simulink model "Combined_Pade_Model_D"  (R2020b)
settings: Solver=VariableStepAuto  StartTime=0.0  StopTime=t_final  MaxStep=0.1  RelTol=1e-3
values from neighbouring files (symbols this model uses):
  c = evalin('base','c')    [output_T.m]    (also in output_V.m; state_eqns_combined_2_n.m; state_eqns_combined_3_n.m; state_eqns_combined_4_n.m)
  p2 = evalin('base','p2')    [output_C_2.m]    (also in state_eqns_combined_2_n.m; state_eqns_combined_2_p.m)
  p3 = evalin('base','p3')    [output_C_3.m]    (also in state_eqns_combined_3_n.m; state_eqns_combined_3_p.m)
  p4 = evalin('base','p4')    [output_C_4.m]    (also in state_eqns_combined_4_n.m; state_eqns_combined_4_p.m)
  p5 = evalin('base','p5')    [output_C_5.m]    (also in state_eqns_combined_5_n.m; state_eqns_combined_5_p.m)
  p6 = evalin('base','p6')    [output_C_6.m]    (also in state_eqns_combined_6_n.m; state_eqns_combined_6_p.m)
  x1n_initial = 0    [Combined_Run_Model.m]
  x2n_initial = 0    [Combined_Run_Model.m]
  x2p_initial = 0    [Combined_Run_Model.m]
  x3n_initial = 0    [Combined_Run_Model.m]
  x3p_initial = 0    [Combined_Run_Model.m]
  x4n_initial = 0    [Combined_Run_Model.m]
  x4p_initial = 0    [Combined_Run_Model.m]
  x5n_initial = 0    [Combined_Run_Model.m]
  x5p_initial = 0    [Combined_Run_Model.m]
  x6n_initial = 0    [Combined_Run_Model.m]
  x6p_initial = 0    [Combined_Run_Model.m]
settings Model: Creator=moonjihoon  LastModifiedBy=moonjihoon

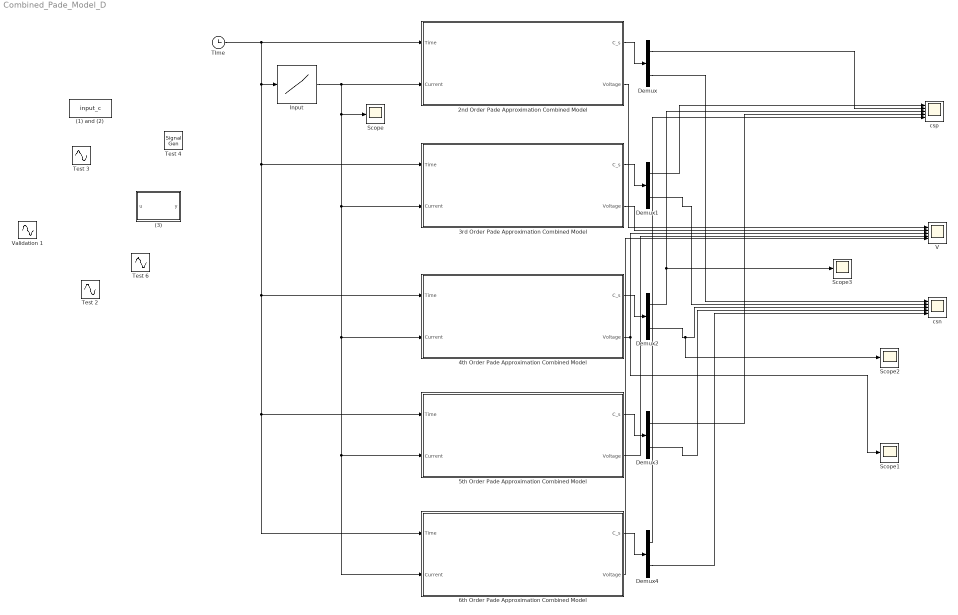
== system Combined_Pade_Model_D ==
  (1) and (2) : MATLABFcn  MATLABFcn=input_c
  (3) : MATLAB Function  TreatAsAtomicUnit=on
  2nd Order Pade Approximation Combined Model : Subsystem
  3rd Order Pade Approximation Combined Model : Subsystem
  4th Order Pade Approximation Combined Model : Subsystem
  5th Order Pade Approximation Combined Model : Subsystem
  6th Order Pade Approximation Combined Model : Subsystem
  Demux{,1..4} (5 alike) : Demux  Outputs=2
  Input : Lookup_n-D  NumberOfTableDimensions=1  BreakpointsForDimension1=t  Table=u  InternalRulePriority=Speed  RndMeth=Simplest  InputSameDT=on
  Scope{,1..3} (4 alike) : Scope
  TIme : Clock
  Test 2 : Sin  Amplitude=10  Frequency=0.005  Phase=3*pi/2  SampleTime=0
  Test 3 : Sin  Amplitude=6  Frequency=0.03  Phase=3*pi/2  SampleTime=0
  Test 4 : SignalGenerator  WaveForm=square  Amplitude=-4  Frequency=0.006  Units=rad/sec
  Test 6 : Sin  Amplitude=10  Frequency=0.005  SampleTime=0
  V : Scope  NumInputPorts=5
  Validation 1 : Sin  Amplitude=5  Frequency=0.02  SampleTime=0
  csn : Scope  NumInputPorts=5
  csp : Scope  NumInputPorts=5
  wires:
  TIme/1 -> Input/1, 6th Order Pade Approximation Combined Model/1(Time), 5th Order Pade Approximation Combined Model/1(Time), 4th Order Pade Approximation Combined Model/1(Time), 3rd Order Pade Approximation Combined Model/1(Time), 2nd Order Pade Approximation Combined Model/1(Time)
  Demux/2 -> csn/1
  Demux/1 -> csp/2
  2nd Order Pade Approximation Combined Model/1(C_s) -> Demux/1
  3rd Order Pade Approximation Combined Model/1(C_s) -> Demux1/1
  Demux1/2 -> csn/2
  Demux1/1 -> csp/1
  Input/1 -> Scope/1, 6th Order Pade Approximation Combined Model/2(Current), 5th Order Pade Approximation Combined Model/2(Current), 4th Order Pade Approximation Combined Model/2(Current), 3rd Order Pade Approximation Combined Model/2(Current), 2nd Order Pade Approximation Combined Model/2(Current)
  Demux2/2 -> Scope2/1, csn/3
  4th Order Pade Approximation Combined Model/1(C_s) -> Demux2/1
  Demux2/1 -> Scope3/1, csp/3
  Demux3/2 -> csn/4
  Demux3/1 -> csp/4
  5th Order Pade Approximation Combined Model/1(C_s) -> Demux3/1
  Demux4/1 -> csp/5
  Demux4/2 -> csn/5
  6th Order Pade Approximation Combined Model/1(C_s) -> Demux4/1
  2nd Order Pade Approximation Combined Model/2(Voltage) -> V/1
  3rd Order Pade Approximation Combined Model/2(Voltage) -> V/2
  4th Order Pade Approximation Combined Model/2(Voltage) -> Scope1/1, V/3
  5th Order Pade Approximation Combined Model/2(Voltage) -> V/4
  6th Order Pade Approximation Combined Model/2(Voltage) -> V/5

== system Combined_Pade_Model_D/2nd Order Pade Approximation Combined Model ==
  Time : Inport
  Current : Inport  Port=2
  Constant : Constant  Value=c.T_inf
  Negative Electrode1 : Subsystem
  OUtput Voltage : Subsystem
  Positive Electrode : Subsystem
  Surface Concentration1 : Subsystem
  C_s : Outport
  Voltage : Outport  Port=2
  wires:
  Time/1 -> Negative Electrode1/1(Time), OUtput Voltage/1(TIme), Surface Concentration1/1(TIme), Positive Electrode/1(TIme)
  Positive Electrode/1(X1,p) -> Surface Concentration1/2(X1,p)
  Positive Electrode/2(X2,p) -> Surface Concentration1/3(X2,p)
  Negative Electrode1/1(X1,n) -> Surface Concentration1/4(X1,n)
  Surface Concentration1/1(C_s) -> OUtput Voltage/3(C_s), C_s/1
  Negative Electrode1/2(X2,n) -> Surface Concentration1/5(X2,n)
  Current/1 -> Negative Electrode1/2(Current), OUtput Voltage/2(Current), Positive Electrode/2(Current)
  Negative Electrode1/3(x2_dot) -> Surface Concentration1/6(X2_dot)
  OUtput Voltage/1(Voltage) -> Voltage/1
  Constant/1 -> OUtput Voltage/4(T)

== system Combined_Pade_Model_D/3rd Order Pade Approximation Combined Model ==
  Time : Inport
  Current : Inport  Port=2
  Constant : Constant  Value=c.T_inf
  Negative Electrode : Subsystem
  OUtput Voltage : Subsystem
  Positive Electrode : Subsystem
  Surface Concentration1 : Subsystem
  C_s : Outport
  Voltage : Outport  Port=2
  wires:
  Time/1 -> OUtput Voltage/1(TIme), Negative Electrode/1(Time), Surface Concentration1/1(TIme), Positive Electrode/1(TIme)
  Current/1 -> Negative Electrode/2(Current), OUtput Voltage/2(Current), Positive Electrode/2(Current)
  Positive Electrode/1(X1,p) -> Surface Concentration1/2(X1,p)
  Positive Electrode/2(X2,p) -> Surface Concentration1/3(X2,p)
  Surface Concentration1/1(C_s) -> OUtput Voltage/3(C_s), C_s/1
  Positive Electrode/3(X3,p) -> Surface Concentration1/4(X3,p)
  Negative Electrode/1(X1,n) -> Surface Concentration1/5(X1,n)
  Negative Electrode/2(X2,n) -> Surface Concentration1/6(X2,n)
  Negative Electrode/3(X3,n) -> Surface Concentration1/7(X3,n)
  Negative Electrode/4(x3_dot) -> Surface Concentration1/8(X3_dot)
  OUtput Voltage/1(Voltage) -> Voltage/1
  Constant/1 -> OUtput Voltage/4(T)

== system Combined_Pade_Model_D/4th Order Pade Approximation Combined Model ==
  Time : Inport
  Current : Inport  Port=2
  Constant : Constant  Value=c.T_inf
  Negative Electrode : Subsystem
  OUtput Voltage : Subsystem
  Positive Electrode : Subsystem
  Surface Concentration1 : Subsystem
  C_s : Outport
  Voltage : Outport  Port=2
  wires:
  Time/1 -> Negative Electrode/1(Time), Positive Electrode/1(TIme), Surface Concentration1/1(TIme), OUtput Voltage/1(TIme)
  Current/1 -> OUtput Voltage/2(Current), Negative Electrode/2(Current), Positive Electrode/2(Current)
  Positive Electrode/1(X1,p) -> Surface Concentration1/2(X1,p)
  Positive Electrode/2(X2,p) -> Surface Concentration1/3(X2,p)
  Surface Concentration1/1(C_s) -> OUtput Voltage/3(C_s), C_s/1
  Positive Electrode/3(X3,p) -> Surface Concentration1/4(X3,p)
  Negative Electrode/5(x4_dot) -> Surface Concentration1/10(X4_dot)
  Positive Electrode/4(X4,p) -> Surface Concentration1/5(X4,p)
  Negative Electrode/1(X1,n) -> Surface Concentration1/6(X1,n)
  Negative Electrode/2(X2,n) -> Surface Concentration1/7(X2,n)
  Negative Electrode/3(X3,n) -> Surface Concentration1/8(X3,n)
  Negative Electrode/4(X4,n) -> Surface Concentration1/9(X4,n)
  OUtput Voltage/1(Voltage) -> Voltage/1
  Constant/1 -> OUtput Voltage/4(T)

== system Combined_Pade_Model_D/5th Order Pade Approximation Combined Model ==
  Time : Inport
  Current : Inport  Port=2
  Constant : Constant  Value=c.T_inf
  Negative Electrode : Subsystem
  OUtput Voltage : Subsystem
  Positive Electrode : Subsystem
  Surface Concentration1 : Subsystem
  C_s : Outport
  Voltage : Outport  Port=2
  wires:
  Time/1 -> Negative Electrode/1(Time), Positive Electrode/1(TIme), OUtput Voltage/1(TIme), Surface Concentration1/1(TIme)
  Current/1 -> Negative Electrode/2(Current), OUtput Voltage/2(Current), Positive Electrode/2(Current)
  Positive Electrode/1(X1,p) -> Surface Concentration1/2(X1,p)
  Positive Electrode/2(X2,p) -> Surface Concentration1/3(X2,p)
  Surface Concentration1/1(C_s) -> OUtput Voltage/3(C_s), C_s/1
  Positive Electrode/3(X3,p) -> Surface Concentration1/4(X3,p)
  Positive Electrode/4(X4,p) -> Surface Concentration1/5(X4,p)
  Positive Electrode/5(X5,p) -> Surface Concentration1/6(X5,p)
  Negative Electrode/1(X1,n) -> Surface Concentration1/7(X1,n)
  Negative Electrode/2(X2,n) -> Surface Concentration1/8(X2,n)
  Negative Electrode/3(X3,n) -> Surface Concentration1/9(X3,n)
  Negative Electrode/4(X4,n) -> Surface Concentration1/10(X4,n)
  Negative Electrode/5(X5,n) -> Surface Concentration1/11(X5,n)
  Negative Electrode/6(x5_dot) -> Surface Concentration1/12(X5_dot)
  OUtput Voltage/1(Voltage) -> Voltage/1
  Constant/1 -> OUtput Voltage/4(T)

== system Combined_Pade_Model_D/6th Order Pade Approximation Combined Model ==
  Time : Inport
  Current : Inport  Port=2
  Constant : Constant  Value=c.T_inf
  Negative Electrode : Subsystem
  OUtput Voltage : Subsystem
  Positive Electrode : Subsystem
  Surface Concentration1 : Subsystem
  C_s : Outport
  Voltage : Outport  Port=2
  wires:
  Time/1 -> Negative Electrode/1(Time), Positive Electrode/1(TIme), OUtput Voltage/1(TIme), Surface Concentration1/1(TIme)
  Current/1 -> OUtput Voltage/2(Current), Negative Electrode/2(Current), Positive Electrode/2(Current)
  Positive Electrode/1(X1,p) -> Surface Concentration1/2(X1,p)
  Positive Electrode/2(X2,p) -> Surface Concentration1/3(X2,p)
  Surface Concentration1/1(C_s) -> OUtput Voltage/3(C_s), C_s/1
  Positive Electrode/3(X3,p) -> Surface Concentration1/4(X3,p)
  Positive Electrode/4(X4,p) -> Surface Concentration1/5(X4,p)
  Positive Electrode/5(X5,p) -> Surface Concentration1/6(X5,p)
  Negative Electrode/1(X1,n) -> Surface Concentration1/8(X1,n)
  Negative Electrode/2(X2,n) -> Surface Concentration1/9(X2,n)
  Negative Electrode/3(X3,n) -> Surface Concentration1/10(X3,n)
  Negative Electrode/4(X4,n) -> Surface Concentration1/11(X4,n)
  Negative Electrode/5(X5,n) -> Surface Concentration1/12(X5,n)
  Negative Electrode/7(x6_dot) -> Surface Concentration1/14(X6_dot)
  Negative Electrode/6(X6,n) -> Surface Concentration1/13(X6,n)
  Positive Electrode/6(X6,p) -> Surface Concentration1/7(X6,p)
  OUtput Voltage/1(Voltage) -> Voltage/1
  Constant/1 -> OUtput Voltage/4(T)

== system Combined_Pade_Model_D/2nd Order Pade Approximation Combined Model/Negative Electrode1 ==
  Time : Inport
  Current : Inport  Port=2
  Dynamics : Subsystem
  X1,n : Outport
  X2,n : Outport  Port=2
  x2_dot : Outport  Port=3
  wires:
  Time/1 -> Dynamics/1(Time)
  Current/1 -> Dynamics/2(Current)
  Dynamics/1(X1,n) -> X1,n/1
  Dynamics/2(X2,n) -> X2,n/1
  Dynamics/3(x2_dot) -> x2_dot/1

== system Combined_Pade_Model_D/2nd Order Pade Approximation Combined Model/OUtput Voltage ==
  TIme : Inport
  Current : Inport  Port=2
  C_s : Inport  Port=3
  T : Inport  Port=4
  Interpreted MATLAB Function : MATLABFcn  MATLABFcn=output_V
  Mux : Mux
  Voltage : Outport
  wires:
  TIme/1 -> Mux/1
  Interpreted MATLAB Function/1 -> Voltage/1
  Mux/1 -> Interpreted MATLAB Function/1
  Current/1 -> Mux/2
  C_s/1 -> Mux/3
  T/1 -> Mux/4

== system Combined_Pade_Model_D/2nd Order Pade Approximation Combined Model/Positive Electrode ==
  TIme : Inport
  Current : Inport  Port=2
  Dynamics : Subsystem
  X1,p : Outport
  X2,p : Outport  Port=2
  wires:
  Current/1 -> Dynamics/2(Current)
  TIme/1 -> Dynamics/1(Time)
  Dynamics/1(X1,p) -> X1,p/1
  Dynamics/2(X2,p) -> X2,p/1

== system Combined_Pade_Model_D/2nd Order Pade Approximation Combined Model/Surface Concentration1 ==
  TIme : Inport
  X1,p : Inport  Port=2
  X2,p : Inport  Port=3
  X1,n : Inport  Port=4
  X2,n : Inport  Port=5
  X2_dot : Inport  Port=6
  Interpreted MATLAB Function : MATLABFcn  MATLABFcn=output_C_2
  Mux : Mux  Inputs=6
  C_s : Outport
  wires:
  Interpreted MATLAB Function/1 -> C_s/1
  Mux/1 -> Interpreted MATLAB Function/1
  X2,p/1 -> Mux/3
  TIme/1 -> Mux/1
  X1,p/1 -> Mux/2
  X1,n/1 -> Mux/4
  X2,n/1 -> Mux/5
  X2_dot/1 -> Mux/6

== system Combined_Pade_Model_D/3rd Order Pade Approximation Combined Model/Negative Electrode ==
  Time : Inport
  Current : Inport  Port=2
  Dynamics : Subsystem
  X1,n : Outport
  X2,n : Outport  Port=2
  X3,n : Outport  Port=3
  x3_dot : Outport  Port=4
  wires:
  Time/1 -> Dynamics/1(Time)
  Current/1 -> Dynamics/2(Current)
  Dynamics/1(X1,n) -> X1,n/1
  Dynamics/2(X2,n) -> X2,n/1
  Dynamics/3(X2,n1) -> X3,n/1
  Dynamics/4(x3_dot) -> x3_dot/1

== system Combined_Pade_Model_D/3rd Order Pade Approximation Combined Model/OUtput Voltage ==
  TIme : Inport
  Current : Inport  Port=2
  C_s : Inport  Port=3
  T : Inport  Port=4
  Interpreted MATLAB Function : MATLABFcn  MATLABFcn=output_V
  Mux : Mux
  Voltage : Outport
  wires:
  TIme/1 -> Mux/1
  Interpreted MATLAB Function/1 -> Voltage/1
  Mux/1 -> Interpreted MATLAB Function/1
  Current/1 -> Mux/2
  C_s/1 -> Mux/3
  T/1 -> Mux/4

== system Combined_Pade_Model_D/3rd Order Pade Approximation Combined Model/Positive Electrode ==
  TIme : Inport
  Current : Inport  Port=2
  Dynamics : Subsystem
  X1,p : Outport
  X2,p : Outport  Port=2
  X3,p : Outport  Port=3
  wires:
  Current/1 -> Dynamics/2(Current)
  TIme/1 -> Dynamics/1(Time)
  Dynamics/1(X1,p) -> X1,p/1
  Dynamics/2(X2,p) -> X2,p/1
  Dynamics/3(X3,p) -> X3,p/1

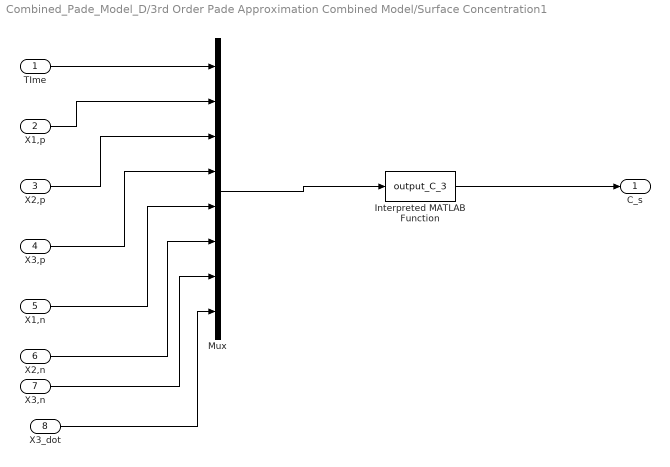
== system Combined_Pade_Model_D/3rd Order Pade Approximation Combined Model/Surface Concentration1 ==
  TIme : Inport
  X1,p : Inport  Port=2
  X2,p : Inport  Port=3
  X3,p : Inport  Port=4
  X1,n : Inport  Port=5
  X2,n : Inport  Port=6
  X3,n : Inport  Port=7
  X3_dot : Inport  Port=8
  Interpreted MATLAB Function : MATLABFcn  MATLABFcn=output_C_3
  Mux : Mux  Inputs=8
  C_s : Outport
  wires:
  Interpreted MATLAB Function/1 -> C_s/1
  Mux/1 -> Interpreted MATLAB Function/1
  X2,p/1 -> Mux/3
  TIme/1 -> Mux/1
  X1,p/1 -> Mux/2
  X3,p/1 -> Mux/4
  X1,n/1 -> Mux/5
  X2,n/1 -> Mux/6
  X3,n/1 -> Mux/7
  X3_dot/1 -> Mux/8

== system Combined_Pade_Model_D/4th Order Pade Approximation Combined Model/Negative Electrode ==
  Time : Inport
  Current : Inport  Port=2
  Dynamics : Subsystem
  X1,n : Outport
  X2,n : Outport  Port=2
  X3,n : Outport  Port=3
  X4,n : Outport  Port=4
  x4_dot : Outport  Port=5
  wires:
  Time/1 -> Dynamics/1(Time)
  Current/1 -> Dynamics/2(Current)
  Dynamics/1(X1,n) -> X1,n/1
  Dynamics/2(X2,n) -> X2,n/1
  Dynamics/3(X3,n) -> X3,n/1
  Dynamics/5(x4_dot) -> x4_dot/1
  Dynamics/4(X4,n) -> X4,n/1

== system Combined_Pade_Model_D/4th Order Pade Approximation Combined Model/OUtput Voltage ==
  TIme : Inport
  Current : Inport  Port=2
  C_s : Inport  Port=3
  T : Inport  Port=4
  Interpreted MATLAB Function : MATLABFcn  MATLABFcn=output_V
  Mux : Mux
  Voltage : Outport
  wires:
  TIme/1 -> Mux/1
  Interpreted MATLAB Function/1 -> Voltage/1
  Mux/1 -> Interpreted MATLAB Function/1
  Current/1 -> Mux/2
  C_s/1 -> Mux/3
  T/1 -> Mux/4

== system Combined_Pade_Model_D/4th Order Pade Approximation Combined Model/Positive Electrode ==
  TIme : Inport
  Current : Inport  Port=2
  Dynamics : Subsystem
  X1,p : Outport
  X2,p : Outport  Port=2
  X3,p : Outport  Port=3
  X4,p : Outport  Port=4
  wires:
  Current/1 -> Dynamics/2(Current)
  TIme/1 -> Dynamics/1(Time)
  Dynamics/1(X1,p) -> X1,p/1
  Dynamics/2(X2,p) -> X2,p/1
  Dynamics/3(X3,p) -> X3,p/1
  Dynamics/4(X4,p) -> X4,p/1

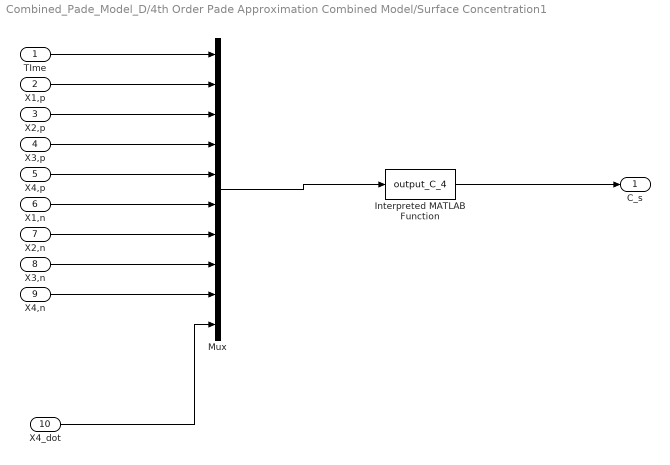
== system Combined_Pade_Model_D/4th Order Pade Approximation Combined Model/Surface Concentration1 ==
  TIme : Inport
  X1,p : Inport  Port=2
  X2,p : Inport  Port=3
  X3,p : Inport  Port=4
  X4,p : Inport  Port=5
  X1,n : Inport  Port=6
  X2,n : Inport  Port=7
  X3,n : Inport  Port=8
  X4,n : Inport  Port=9
  X4_dot : Inport  Port=10
  Interpreted MATLAB Function : MATLABFcn  MATLABFcn=output_C_4
  Mux : Mux  Inputs=10
  C_s : Outport
  wires:
  Interpreted MATLAB Function/1 -> C_s/1
  Mux/1 -> Interpreted MATLAB Function/1
  X2,p/1 -> Mux/3
  TIme/1 -> Mux/1
  X1,p/1 -> Mux/2
  X3,p/1 -> Mux/4
  X4,p/1 -> Mux/5
  X1,n/1 -> Mux/6
  X2,n/1 -> Mux/7
  X4_dot/1 -> Mux/10
  X3,n/1 -> Mux/8
  X4,n/1 -> Mux/9

== system Combined_Pade_Model_D/5th Order Pade Approximation Combined Model/Negative Electrode ==
  Time : Inport
  Current : Inport  Port=2
  Dynamics : Subsystem
  X1,n : Outport
  X2,n : Outport  Port=2
  X3,n : Outport  Port=3
  X4,n : Outport  Port=4
  X5,n : Outport  Port=5
  x5_dot : Outport  Port=6
  wires:
  Time/1 -> Dynamics/1(Time)
  Current/1 -> Dynamics/2(Current)
  Dynamics/1(X1,n) -> X1,n/1
  Dynamics/2(X2,n) -> X2,n/1
  Dynamics/3(X3,n) -> X3,n/1
  Dynamics/6(x5_dot) -> x5_dot/1
  Dynamics/4(X4,n) -> X4,n/1
  Dynamics/5(X5,n) -> X5,n/1

== system Combined_Pade_Model_D/5th Order Pade Approximation Combined Model/OUtput Voltage ==
  TIme : Inport
  Current : Inport  Port=2
  C_s : Inport  Port=3
  T : Inport  Port=4
  Interpreted MATLAB Function : MATLABFcn  MATLABFcn=output_V
  Mux : Mux
  Voltage : Outport
  wires:
  TIme/1 -> Mux/1
  Interpreted MATLAB Function/1 -> Voltage/1
  Mux/1 -> Interpreted MATLAB Function/1
  Current/1 -> Mux/2
  C_s/1 -> Mux/3
  T/1 -> Mux/4

== system Combined_Pade_Model_D/5th Order Pade Approximation Combined Model/Positive Electrode ==
  TIme : Inport
  Current : Inport  Port=2
  Dynamics : Subsystem
  X1,p : Outport
  X2,p : Outport  Port=2
  X3,p : Outport  Port=3
  X4,p : Outport  Port=4
  X5,p : Outport  Port=5
  wires:
  Current/1 -> Dynamics/2(Current)
  TIme/1 -> Dynamics/1(Time)
  Dynamics/1(X1,p) -> X1,p/1
  Dynamics/2(X2,p) -> X2,p/1
  Dynamics/3(X3,p) -> X3,p/1
  Dynamics/4(X4,p) -> X4,p/1
  Dynamics/5(X5,p) -> X5,p/1

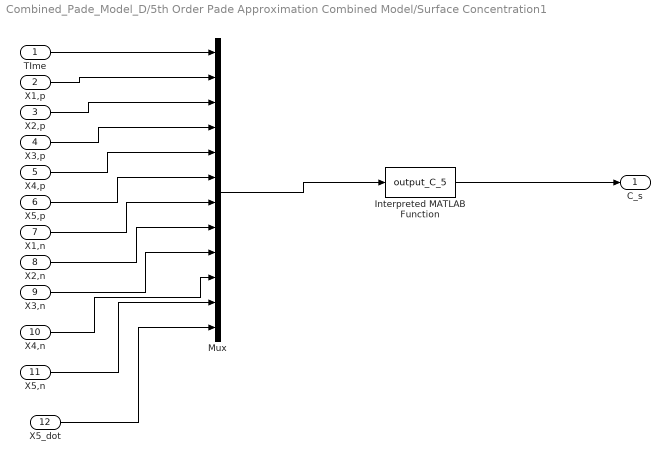
== system Combined_Pade_Model_D/5th Order Pade Approximation Combined Model/Surface Concentration1 ==
  TIme : Inport
  X1,p : Inport  Port=2
  X2,p : Inport  Port=3
  X3,p : Inport  Port=4
  X4,p : Inport  Port=5
  X5,p : Inport  Port=6
  X1,n : Inport  Port=7
  X2,n : Inport  Port=8
  X3,n : Inport  Port=9
  X4,n : Inport  Port=10
  X5,n : Inport  Port=11
  X5_dot : Inport  Port=12
  Interpreted MATLAB Function : MATLABFcn  MATLABFcn=output_C_5
  Mux : Mux  Inputs=12
  C_s : Outport
  wires:
  Interpreted MATLAB Function/1 -> C_s/1
  Mux/1 -> Interpreted MATLAB Function/1
  X2,p/1 -> Mux/3
  TIme/1 -> Mux/1
  X1,p/1 -> Mux/2
  X3,p/1 -> Mux/4
  X4,p/1 -> Mux/5
  X5,p/1 -> Mux/6
  X1,n/1 -> Mux/7
  X2,n/1 -> Mux/8
  X3,n/1 -> Mux/9
  X5_dot/1 -> Mux/12
  X4,n/1 -> Mux/10
  X5,n/1 -> Mux/11

== system Combined_Pade_Model_D/6th Order Pade Approximation Combined Model/Negative Electrode ==
  Time : Inport
  Current : Inport  Port=2
  Dynamics : Subsystem
  X1,n : Outport
  X2,n : Outport  Port=2
  X3,n : Outport  Port=3
  X4,n : Outport  Port=4
  X5,n : Outport  Port=5
  X6,n : Outport  Port=6
  x6_dot : Outport  Port=7
  wires:
  Time/1 -> Dynamics/1(Time)
  Current/1 -> Dynamics/2(Current)
  Dynamics/1(X1,n) -> X1,n/1
  Dynamics/2(X2,n) -> X2,n/1
  Dynamics/3(X3,n) -> X3,n/1
  Dynamics/7(x6_dot) -> x6_dot/1
  Dynamics/4(X4,n) -> X4,n/1
  Dynamics/5(X5,n) -> X5,n/1
  Dynamics/6(X6,n) -> X6,n/1

== system Combined_Pade_Model_D/6th Order Pade Approximation Combined Model/OUtput Voltage ==
  TIme : Inport
  Current : Inport  Port=2
  C_s : Inport  Port=3
  T : Inport  Port=4
  Interpreted MATLAB Function : MATLABFcn  MATLABFcn=output_V
  Mux : Mux
  Voltage : Outport
  wires:
  TIme/1 -> Mux/1
  Interpreted MATLAB Function/1 -> Voltage/1
  Mux/1 -> Interpreted MATLAB Function/1
  Current/1 -> Mux/2
  C_s/1 -> Mux/3
  T/1 -> Mux/4

== system Combined_Pade_Model_D/6th Order Pade Approximation Combined Model/Positive Electrode ==
  TIme : Inport
  Current : Inport  Port=2
  Dynamics : Subsystem
  X1,p : Outport
  X2,p : Outport  Port=2
  X3,p : Outport  Port=3
  X4,p : Outport  Port=4
  X5,p : Outport  Port=5
  X6,p : Outport  Port=6
  wires:
  Current/1 -> Dynamics/2(Current)
  TIme/1 -> Dynamics/1(Time)
  Dynamics/1(X1,p) -> X1,p/1
  Dynamics/2(X2,p) -> X2,p/1
  Dynamics/3(X3,p) -> X3,p/1
  Dynamics/4(X4,p) -> X4,p/1
  Dynamics/5(X5,p) -> X5,p/1
  Dynamics/6(X6,p) -> X6,p/1

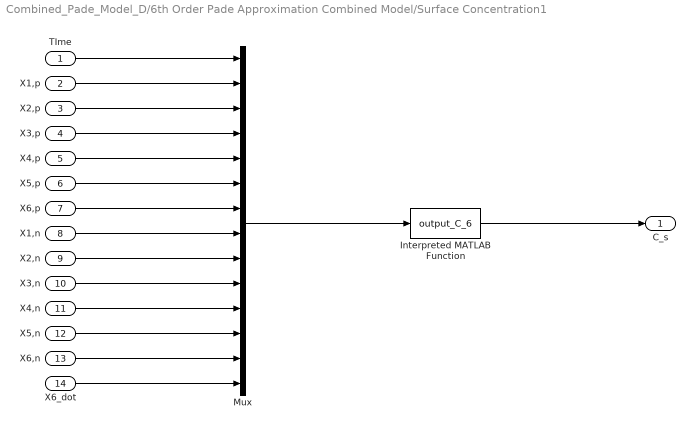
== system Combined_Pade_Model_D/6th Order Pade Approximation Combined Model/Surface Concentration1 ==
  TIme : Inport
  X1,p : Inport  Port=2
  X2,p : Inport  Port=3
  X3,p : Inport  Port=4
  X4,p : Inport  Port=5
  X5,p : Inport  Port=6
  X6,p : Inport  Port=7
  X1,n : Inport  Port=8
  X2,n : Inport  Port=9
  X3,n : Inport  Port=10
  X4,n : Inport  Port=11
  X5,n : Inport  Port=12
  X6,n : Inport  Port=13
  X6_dot : Inport  Port=14
  Interpreted MATLAB Function : MATLABFcn  MATLABFcn=output_C_6
  Mux : Mux  Inputs=14
  C_s : Outport
  wires:
  Interpreted MATLAB Function/1 -> C_s/1
  Mux/1 -> Interpreted MATLAB Function/1
  X6_dot/1 -> Mux/14
  TIme/1 -> Mux/1
  X1,p/1 -> Mux/2
  X2,p/1 -> Mux/3
  X3,p/1 -> Mux/4
  X4,p/1 -> Mux/5
  X5,p/1 -> Mux/6
  X6,p/1 -> Mux/7
  X1,n/1 -> Mux/8
  X2,n/1 -> Mux/9
  X3,n/1 -> Mux/10
  X4,n/1 -> Mux/11
  X5,n/1 -> Mux/12
  X6,n/1 -> Mux/13

== system Combined_Pade_Model_D/2nd Order Pade Approximation Combined Model/Negative Electrode1/Dynamics ==
  Time : Inport
  Current : Inport  Port=2
  Integrator : Integrator  InitialCondition=[x1n_initial;x2n_initial]
  Interpreted MATLAB Function : MATLABFcn  MATLABFcn=state_eqns_combined_2_n
  Mux : Mux  Inputs=3
  Selector : Selector  InputPortWidth=2  IndexOptions=Index vector (dialog)  Indices=[1]  OutputSizes=1
  Selector1 : Selector  InputPortWidth=2  IndexOptions=Index vector (dialog)  Indices=[2]  OutputSizes=1
  X1,n : Outport
  X2,n : Outport  Port=2
  x2_dot : Outport  Port=3
  wires:
  Current/1 -> Mux/2
  Time/1 -> Mux/1
  Selector/1 -> X1,n/1
  Selector1/1 -> X2,n/1
  Mux/1 -> Interpreted MATLAB Function/1
  Integrator/1 -> Mux/3, Selector1/1, Selector/1
  Interpreted MATLAB Function/1 -> x2_dot/1, Integrator/1

== system Combined_Pade_Model_D/2nd Order Pade Approximation Combined Model/Positive Electrode/Dynamics ==
  Time : Inport
  Current : Inport  Port=2
  Integrator : Integrator  InitialCondition=[p2.x1p_initial;x2p_initial]
  Interpreted MATLAB Function : MATLABFcn  MATLABFcn=state_eqns_combined_2_p
  Mux : Mux  Inputs=3
  Selector : Selector  InputPortWidth=2  IndexOptions=Index vector (dialog)  Indices=[1]  OutputSizes=1
  Selector1 : Selector  InputPortWidth=2  IndexOptions=Index vector (dialog)  Indices=[2]  OutputSizes=1
  X1,p : Outport
  X2,p : Outport  Port=2
  wires:
  Current/1 -> Mux/2
  Time/1 -> Mux/1
  Interpreted MATLAB Function/1 -> Integrator/1
  Selector/1 -> X1,p/1
  Selector1/1 -> X2,p/1
  Mux/1 -> Interpreted MATLAB Function/1
  Integrator/1 -> Mux/3, Selector1/1, Selector/1

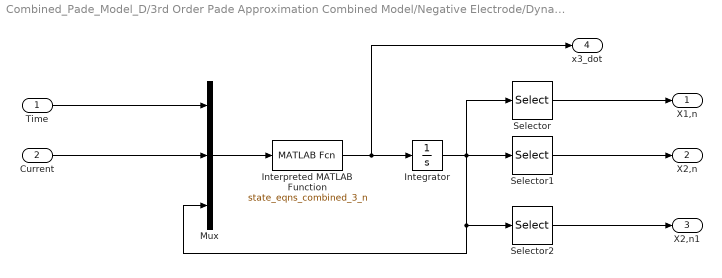
== system Combined_Pade_Model_D/3rd Order Pade Approximation Combined Model/Negative Electrode/Dynamics ==
  Time : Inport
  Current : Inport  Port=2
  Integrator : Integrator  InitialCondition=[x1n_initial;x2n_initial;x3n_initial]
  Interpreted MATLAB Function : MATLABFcn  MATLABFcn=state_eqns_combined_3_n
  Mux : Mux  Inputs=3
  Selector : Selector  InputPortWidth=3  IndexOptions=Index vector (dialog)  Indices=[1]  OutputSizes=1
  Selector1 : Selector  InputPortWidth=3  IndexOptions=Index vector (dialog)  Indices=[2]  OutputSizes=1
  Selector2 : Selector  InputPortWidth=3  IndexOptions=Index vector (dialog)  Indices=[3]  OutputSizes=1
  X1,n : Outport
  X2,n : Outport  Port=2
  X2,n1 : Outport  Port=3
  x3_dot : Outport  Port=4
  wires:
  Current/1 -> Mux/2
  Time/1 -> Mux/1
  Selector/1 -> X1,n/1
  Selector1/1 -> X2,n/1
  Mux/1 -> Interpreted MATLAB Function/1
  Selector2/1 -> X2,n1/1
  Integrator/1 -> Selector2/1, Mux/3, Selector1/1, Selector/1
  Interpreted MATLAB Function/1 -> x3_dot/1, Integrator/1

== system Combined_Pade_Model_D/3rd Order Pade Approximation Combined Model/Positive Electrode/Dynamics ==
  Time : Inport
  Current : Inport  Port=2
  Integrator : Integrator  InitialCondition=[p3.x1p_initial;x2p_initial;x3p_initial]
  Interpreted MATLAB Function : MATLABFcn  MATLABFcn=state_eqns_combined_3_p
  Mux : Mux  Inputs=3
  Selector : Selector  InputPortWidth=3  IndexOptions=Index vector (dialog)  Indices=[1]  OutputSizes=1
  Selector1 : Selector  InputPortWidth=3  IndexOptions=Index vector (dialog)  Indices=[2]  OutputSizes=1
  Selector2 : Selector  InputPortWidth=3  IndexOptions=Index vector (dialog)  Indices=[3]  OutputSizes=1
  X1,p : Outport
  X2,p : Outport  Port=2
  X3,p : Outport  Port=3
  wires:
  Current/1 -> Mux/2
  Time/1 -> Mux/1
  Interpreted MATLAB Function/1 -> Integrator/1
  Selector/1 -> X1,p/1
  Selector1/1 -> X2,p/1
  Mux/1 -> Interpreted MATLAB Function/1
  Integrator/1 -> Selector2/1, Mux/3, Selector1/1, Selector/1
  Selector2/1 -> X3,p/1

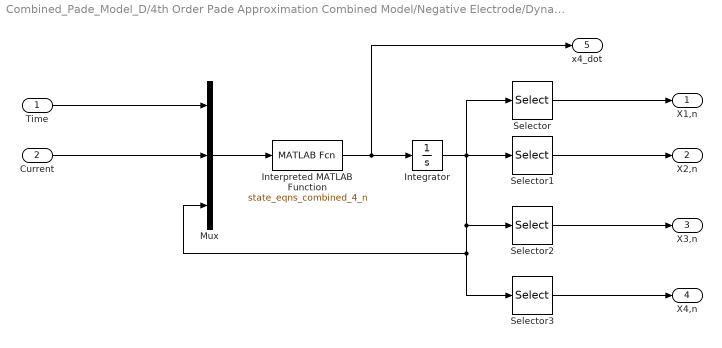
== system Combined_Pade_Model_D/4th Order Pade Approximation Combined Model/Negative Electrode/Dynamics ==
  Time : Inport
  Current : Inport  Port=2
  Integrator : Integrator  InitialCondition=[x1n_initial;x2n_initial;x3n_initial;x4n_initial]
  Interpreted MATLAB Function : MATLABFcn  MATLABFcn=state_eqns_combined_4_n
  Mux : Mux  Inputs=3
  Selector : Selector  InputPortWidth=4  IndexOptions=Index vector (dialog)  Indices=[1]  OutputSizes=1
  Selector1 : Selector  InputPortWidth=4  IndexOptions=Index vector (dialog)  Indices=[2]  OutputSizes=1
  Selector2 : Selector  InputPortWidth=4  IndexOptions=Index vector (dialog)  Indices=[3]  OutputSizes=1
  Selector3 : Selector  InputPortWidth=4  IndexOptions=Index vector (dialog)  Indices=[4]  OutputSizes=1
  X1,n : Outport
  X2,n : Outport  Port=2
  X3,n : Outport  Port=3
  X4,n : Outport  Port=4
  x4_dot : Outport  Port=5
  wires:
  Current/1 -> Mux/2
  Time/1 -> Mux/1
  Selector/1 -> X1,n/1
  Selector1/1 -> X2,n/1
  Mux/1 -> Interpreted MATLAB Function/1
  Selector2/1 -> X3,n/1
  Integrator/1 -> Selector2/1, Selector3/1, Mux/3, Selector1/1, Selector/1
  Interpreted MATLAB Function/1 -> x4_dot/1, Integrator/1
  Selector3/1 -> X4,n/1

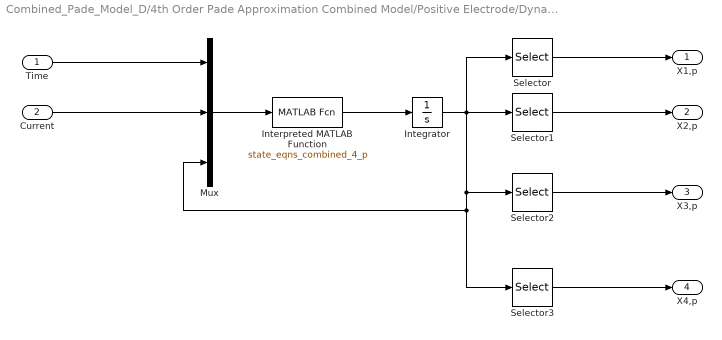
== system Combined_Pade_Model_D/4th Order Pade Approximation Combined Model/Positive Electrode/Dynamics ==
  Time : Inport
  Current : Inport  Port=2
  Integrator : Integrator  InitialCondition=[p4.x1p_initial;x2p_initial;x3p_initial;x4p_initial]
  Interpreted MATLAB Function : MATLABFcn  MATLABFcn=state_eqns_combined_4_p
  Mux : Mux  Inputs=3
  Selector : Selector  InputPortWidth=4  IndexOptions=Index vector (dialog)  Indices=[1]  OutputSizes=1
  Selector1 : Selector  InputPortWidth=4  IndexOptions=Index vector (dialog)  Indices=[2]  OutputSizes=1
  Selector2 : Selector  InputPortWidth=4  IndexOptions=Index vector (dialog)  Indices=[3]  OutputSizes=1
  Selector3 : Selector  InputPortWidth=4  IndexOptions=Index vector (dialog)  Indices=[4]  OutputSizes=1
  X1,p : Outport
  X2,p : Outport  Port=2
  X3,p : Outport  Port=3
  X4,p : Outport  Port=4
  wires:
  Current/1 -> Mux/2
  Time/1 -> Mux/1
  Interpreted MATLAB Function/1 -> Integrator/1
  Selector/1 -> X1,p/1
  Selector1/1 -> X2,p/1
  Mux/1 -> Interpreted MATLAB Function/1
  Selector2/1 -> X3,p/1
  Selector3/1 -> X4,p/1
  Integrator/1 -> Selector2/1, Selector3/1, Mux/3, Selector1/1, Selector/1

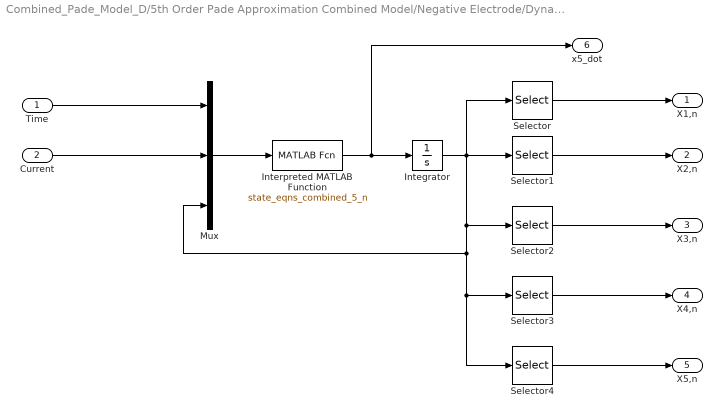
== system Combined_Pade_Model_D/5th Order Pade Approximation Combined Model/Negative Electrode/Dynamics ==
  Time : Inport
  Current : Inport  Port=2
  Integrator : Integrator  InitialCondition=[x1n_initial;x2n_initial;x3n_initial;x4n_initial;x5n_initial]
  Interpreted MATLAB Function : MATLABFcn  MATLABFcn=state_eqns_combined_5_n
  Mux : Mux  Inputs=3
  Selector : Selector  InputPortWidth=5  IndexOptions=Index vector (dialog)  Indices=[1]  OutputSizes=1
  Selector1 : Selector  InputPortWidth=5  IndexOptions=Index vector (dialog)  Indices=[2]  OutputSizes=1
  Selector2 : Selector  InputPortWidth=5  IndexOptions=Index vector (dialog)  Indices=[3]  OutputSizes=1
  Selector3 : Selector  InputPortWidth=5  IndexOptions=Index vector (dialog)  Indices=[4]  OutputSizes=1
  Selector4 : Selector  InputPortWidth=5  IndexOptions=Index vector (dialog)  Indices=[5]  OutputSizes=1
  X1,n : Outport
  X2,n : Outport  Port=2
  X3,n : Outport  Port=3
  X4,n : Outport  Port=4
  X5,n : Outport  Port=5
  x5_dot : Outport  Port=6
  wires:
  Current/1 -> Mux/2
  Time/1 -> Mux/1
  Selector/1 -> X1,n/1
  Selector1/1 -> X2,n/1
  Mux/1 -> Interpreted MATLAB Function/1
  Selector2/1 -> X3,n/1
  Interpreted MATLAB Function/1 -> x5_dot/1, Integrator/1
  Selector3/1 -> X4,n/1
  Selector4/1 -> X5,n/1
  Integrator/1 -> Selector2/1, Selector4/1, Selector3/1, Mux/3, Selector1/1, Selector/1

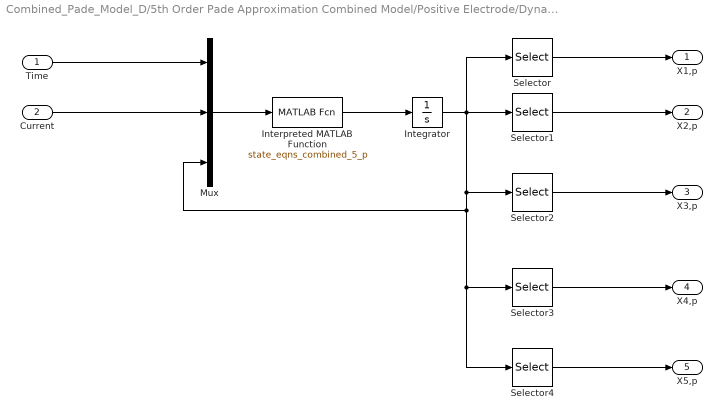
== system Combined_Pade_Model_D/5th Order Pade Approximation Combined Model/Positive Electrode/Dynamics ==
  Time : Inport
  Current : Inport  Port=2
  Integrator : Integrator  InitialCondition=[p5.x1p_initial;x2p_initial;x3p_initial;x4p_initial;x5p_initial]
  Interpreted MATLAB Function : MATLABFcn  MATLABFcn=state_eqns_combined_5_p
  Mux : Mux  Inputs=3
  Selector : Selector  InputPortWidth=5  IndexOptions=Index vector (dialog)  Indices=[1]  OutputSizes=1
  Selector1 : Selector  InputPortWidth=5  IndexOptions=Index vector (dialog)  Indices=[2]  OutputSizes=1
  Selector2 : Selector  InputPortWidth=5  IndexOptions=Index vector (dialog)  Indices=[3]  OutputSizes=1
  Selector3 : Selector  InputPortWidth=5  IndexOptions=Index vector (dialog)  Indices=[4]  OutputSizes=1
  Selector4 : Selector  InputPortWidth=5  IndexOptions=Index vector (dialog)  Indices=[5]  OutputSizes=1
  X1,p : Outport
  X2,p : Outport  Port=2
  X3,p : Outport  Port=3
  X4,p : Outport  Port=4
  X5,p : Outport  Port=5
  wires:
  Current/1 -> Mux/2
  Time/1 -> Mux/1
  Interpreted MATLAB Function/1 -> Integrator/1
  Selector/1 -> X1,p/1
  Selector1/1 -> X2,p/1
  Mux/1 -> Interpreted MATLAB Function/1
  Selector2/1 -> X3,p/1
  Selector3/1 -> X4,p/1
  Selector4/1 -> X5,p/1
  Integrator/1 -> Selector2/1, Selector4/1, Selector3/1, Mux/3, Selector1/1, Selector/1

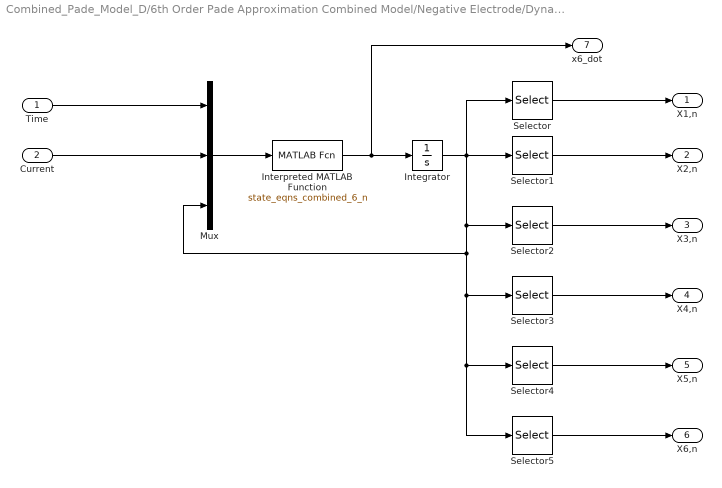
== system Combined_Pade_Model_D/6th Order Pade Approximation Combined Model/Negative Electrode/Dynamics ==
  Time : Inport
  Current : Inport  Port=2
  Integrator : Integrator  InitialCondition=[x1n_initial;x2n_initial;x3n_initial;x4n_initial;x5n_initial;x6n_initial]
  Interpreted MATLAB Function : MATLABFcn  MATLABFcn=state_eqns_combined_6_n
  Mux : Mux  Inputs=3
  Selector : Selector  InputPortWidth=6  IndexOptions=Index vector (dialog)  Indices=[1]  OutputSizes=1
  Selector1 : Selector  InputPortWidth=6  IndexOptions=Index vector (dialog)  Indices=[2]  OutputSizes=1
  Selector2 : Selector  InputPortWidth=6  IndexOptions=Index vector (dialog)  Indices=[3]  OutputSizes=1
  Selector3 : Selector  InputPortWidth=6  IndexOptions=Index vector (dialog)  Indices=[4]  OutputSizes=1
  Selector4 : Selector  InputPortWidth=6  IndexOptions=Index vector (dialog)  Indices=[5]  OutputSizes=1
  Selector5 : Selector  InputPortWidth=6  IndexOptions=Index vector (dialog)  Indices=[6]  OutputSizes=1
  X1,n : Outport
  X2,n : Outport  Port=2
  X3,n : Outport  Port=3
  X4,n : Outport  Port=4
  X5,n : Outport  Port=5
  X6,n : Outport  Port=6
  x6_dot : Outport  Port=7
  wires:
  Current/1 -> Mux/2
  Time/1 -> Mux/1
  Selector/1 -> X1,n/1
  Selector1/1 -> X2,n/1
  Mux/1 -> Interpreted MATLAB Function/1
  Selector2/1 -> X3,n/1
  Interpreted MATLAB Function/1 -> x6_dot/1, Integrator/1
  Selector3/1 -> X4,n/1
  Selector4/1 -> X5,n/1
  Integrator/1 -> Selector2/1, Selector5/1, Selector4/1, Selector3/1, Mux/3, Selector1/1, Selector/1
  Selector5/1 -> X6,n/1

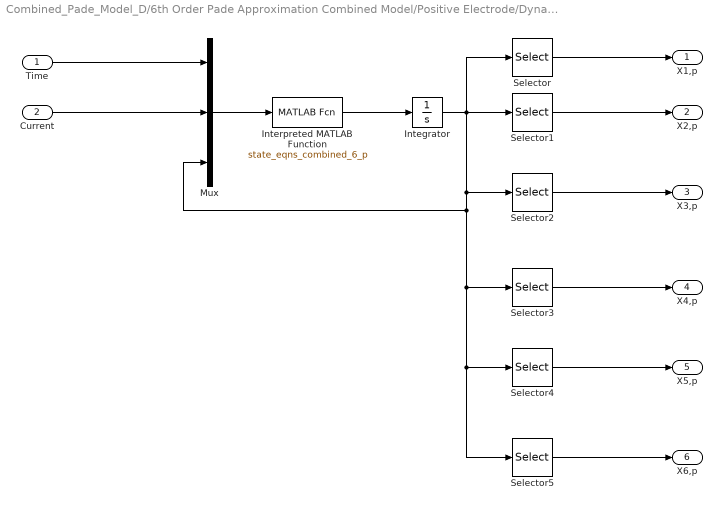
== system Combined_Pade_Model_D/6th Order Pade Approximation Combined Model/Positive Electrode/Dynamics ==
  Time : Inport
  Current : Inport  Port=2
  Integrator : Integrator  InitialCondition=[p6.x1p_initial;x2p_initial;x3p_initial;x4p_initial;x5p_initial;x6p_initial]
  Interpreted MATLAB Function : MATLABFcn  MATLABFcn=state_eqns_combined_6_p
  Mux : Mux  Inputs=3
  Selector : Selector  InputPortWidth=6  IndexOptions=Index vector (dialog)  Indices=[1]  OutputSizes=1
  Selector1 : Selector  InputPortWidth=6  IndexOptions=Index vector (dialog)  Indices=[2]  OutputSizes=1
  Selector2 : Selector  InputPortWidth=6  IndexOptions=Index vector (dialog)  Indices=[3]  OutputSizes=1
  Selector3 : Selector  InputPortWidth=6  IndexOptions=Index vector (dialog)  Indices=[4]  OutputSizes=1
  Selector4 : Selector  InputPortWidth=6  IndexOptions=Index vector (dialog)  Indices=[5]  OutputSizes=1
  Selector5 : Selector  InputPortWidth=6  IndexOptions=Index vector (dialog)  Indices=[6]  OutputSizes=1
  X1,p : Outport
  X2,p : Outport  Port=2
  X3,p : Outport  Port=3
  X4,p : Outport  Port=4
  X5,p : Outport  Port=5
  X6,p : Outport  Port=6
  wires:
  Current/1 -> Mux/2
  Time/1 -> Mux/1
  Interpreted MATLAB Function/1 -> Integrator/1
  Selector/1 -> X1,p/1
  Selector1/1 -> X2,p/1
  Mux/1 -> Interpreted MATLAB Function/1
  Selector2/1 -> X3,p/1
  Selector3/1 -> X4,p/1
  Selector4/1 -> X5,p/1
  Integrator/1 -> Selector2/1, Selector5/1, Selector4/1, Selector3/1, Mux/3, Selector1/1, Selector/1
  Selector5/1 -> X6,p/1

== matlab function Combined_Pade_Model_D/(3) ==
  data: u input; y output
function y = fcn(u)

y = exp(-0.0055*u).*10.*sin(0.02*pi*u);
